simulink model "SignalConditioning_Controller"  (R2021b)
settings: Solver=VariableStepAuto  StartTime=0.0  StopTime=10.0  RelTol=1e-3
settings Model: Creator=matas  LastModifiedBy=matas

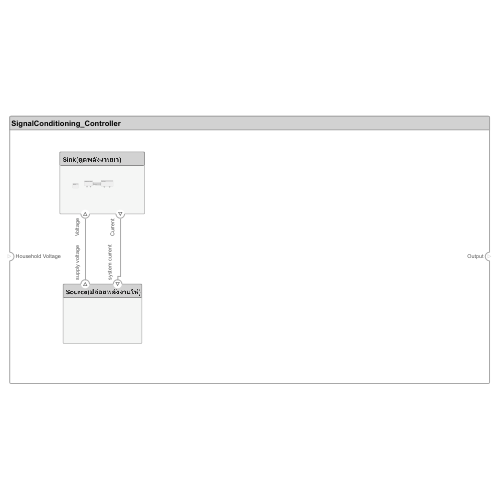
[thumbnail: Simulink's stored preview of the top-level diagram]
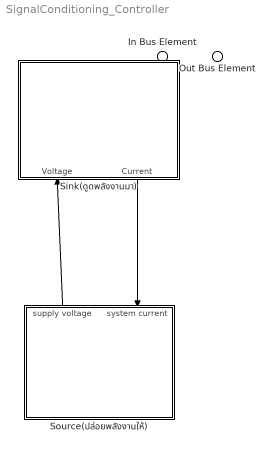
== system SignalConditioning_Controller ==
  In Bus Element : Inport  PortName=Household Voltage
  Sink(ดูดพลังงานมา) : Subsystem
      settings: PortSchema="{\"entries\":[{\"content\":{\"headerSize\":26,\"margin\":15,\"minimumSpacing\":25,\"sides\":[{\"content\":{\"connectorIds\":[]},\"type\":\"ConnectorPlacement.EquallySpacedRectSide\",\"uuid\":\"92879829-3325-4e99-8cb7-644760838beb\"},{\"content\":{\"connectorIds\":[],\"side\":\"RIGHT\"},\"type\":\"ConnectorPlacement.EquallySpacedRectSide\",\"uuid\":\"7f28acab-39b7-45d1-ae7e-3b59846b890e\"},{\"content\":{\"connectorIds\":[],\"side\":\"TOP\"},\"type\":\"ConnectorPlacement.EquallySpacedRectSide\",\"uuid\":\"948d0c2c-a98c-4918-8c8b-513a78882665\"},{\"content\":{\"connectorIds\":[\"In1\",\"Out1\"],\"side\":\"BOTTOM\"},\"type\":\"ConnectorPlacement.EquallySpacedRectSide\",\"uuid\":\"f8beaf20-50aa-47d8-aac6-799df18d83d8\"}]},\"type\":\"ConnectorPlacement.EquallySpacedConnector\",\"uuid\":\"4e812113-efb0-4c93-881b-0cbb00878572\"}],\"packageUris\":[\"http://schema.mathworks.com/mf0/Connector/R2020b\"],\"version\":\"1.0\"}"
  Source(ปล่อยพลังงานให้) : Subsystem
      settings: PortSchema="{\"entries\":[{\"content\":{\"headerSize\":26,\"margin\":15,\"minimumSpacing\":25,\"sides\":[{\"content\":{\"connectorIds\":[]},\"type\":\"ConnectorPlacement.EquallySpacedRectSide\",\"uuid\":\"92879829-3325-4e99-8cb7-644760838beb\"},{\"content\":{\"connectorIds\":[],\"side\":\"RIGHT\"},\"type\":\"ConnectorPlacement.EquallySpacedRectSide\",\"uuid\":\"7f28acab-39b7-45d1-ae7e-3b59846b890e\"},{\"content\":{\"connectorIds\":[\"Out1\",\"In1\"],\"side\":\"TOP\"},\"type\":\"ConnectorPlacement.EquallySpacedRectSide\",\"uuid\":\"948d0c2c-a98c-4918-8c8b-513a78882665\"}]},\"type\":\"ConnectorPlacement.EquallySpacedConnector\",\"uuid\":\"4e812113-efb0-4c93-881b-0cbb00878572\"}],\"packageUris\":[\"http://schema.mathworks.com/mf0/Connector/R2020b\"],\"version\":\"1.0\"}"
  Out Bus Element : Outport  PortName=Output
  wires:
  Source(ปล่อยพลังงานให้)/1(supply voltage) -> Sink(ดูดพลังงานมา)/1(Voltage)
  Sink(ดูดพลังงานมา)/1(Current) -> Source(ปล่อยพลังงานให้)/1(system current)

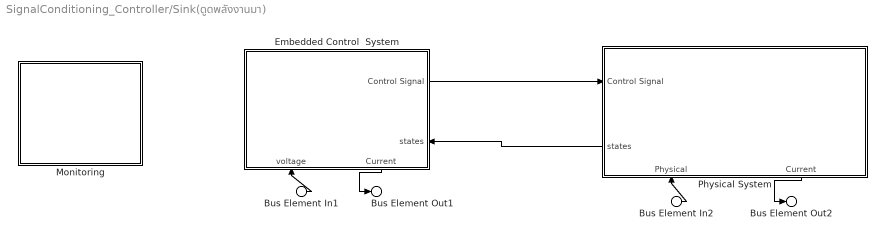
== system SignalConditioning_Controller/Sink(ดูดพลังงานมา) ==
  Bus Element In1 : Inport  PortName=Voltage  Element=Control
  Bus Element In2 : Inport  PortName=Voltage  Element=Physical
  Embedded Control  System : Subsystem
      settings: PortSchema="{\"entries\":[{\"content\":{\"headerSize\":26,\"margin\":15,\"minimumSpacing\":25,\"sides\":[{\"content\":{\"connectorIds\":[]},\"type\":\"ConnectorPlacement.EquallySpacedRectSide\",\"uuid\":\"92879829-3325-4e99-8cb7-644760838beb\"},{\"content\":{\"connectorIds\":[\"Out1\",\"In1\"],\"side\":\"RIGHT\"},\"type\":\"ConnectorPlacement.EquallySpacedRectSide\",\"uuid\":\"7f28acab-39b7-45d1-ae7e-3b59846b890e\"},{\"content\":{\"connectorIds\":[],\"side\":\"TOP\"},\"type\":\"ConnectorPlacement.EquallySpacedRectSide\",\"uuid\":\"948d0c2c-a98c-4918-8c8b-513a78882665\"},{\"content\":{\"connectorIds\":[\"In2\",\"Out2\"],\"side\":\"BOTTOM\"},\"type\":\"ConnectorPlacement.EquallySpacedRectSide\",\"uuid\":\"a92c0028-d905-4fe1-b620-96383c5e960c\"}]},\"type\":\"ConnectorPlacement.EquallySpacedConnector\",\"uuid\":\"4e812113-efb0-4c93-881b-0cbb00878572\"}],\"packageUris\":[\"http://schema.mathworks.com/mf0/Connector/R2020b\"],\"version\":\"1.0\"}"
  Monitoring : Subsystem
      settings: PortSchema="{\"entries\":[{\"content\":{\"headerSize\":26,\"margin\":15,\"minimumSpacing\":25,\"sides\":[{\"content\":{\"connectorIds\":[]},\"type\":\"ConnectorPlacement.EquallySpacedRectSide\",\"uuid\":\"92879829-3325-4e99-8cb7-644760838beb\"},{\"content\":{\"connectorIds\":[],\"side\":\"RIGHT\"},\"type\":\"ConnectorPlacement.EquallySpacedRectSide\",\"uuid\":\"7f28acab-39b7-45d1-ae7e-3b59846b890e\"},{\"content\":{\"connectorIds\":[],\"side\":\"TOP\"},\"type\":\"ConnectorPlacement.EquallySpacedRectSide\",\"uuid\":\"948d0c2c-a98c-4918-8c8b-513a78882665\"}]},\"type\":\"ConnectorPlacement.EquallySpacedConnector\",\"uuid\":\"4e812113-efb0-4c93-881b-0cbb00878572\"}],\"packageUris\":[\"http://schema.mathworks.com/mf0/Connector/R2020b\"],\"version\":\"1.0\"}"
  Physical System : Subsystem
      settings: PortSchema="{\"entries\":[{\"content\":{\"headerSize\":26,\"margin\":15,\"minimumSpacing\":25,\"sides\":[{\"content\":{\"connectorIds\":[\"In1\",\"Out1\"]},\"type\":\"ConnectorPlacement.EquallySpacedRectSide\",\"uuid\":\"92879829-3325-4e99-8cb7-644760838beb\"},{\"content\":{\"connectorIds\":[],\"side\":\"RIGHT\"},\"type\":\"ConnectorPlacement.EquallySpacedRectSide\",\"uuid\":\"7f28acab-39b7-45d1-ae7e-3b59846b890e\"},{\"content\":{\"connectorIds\":[],\"side\":\"TOP\"},\"type\":\"ConnectorPlacement.EquallySpacedRectSide\",\"uuid\":\"948d0c2c-a98c-4918-8c8b-513a78882665\"},{\"content\":{\"connectorIds\":[\"In2\",\"Out2\"],\"side\":\"BOTTOM\"},\"type\":\"ConnectorPlacement.EquallySpacedRectSide\",\"uuid\":\"84b42df1-53ca-4145-9269-aa3d14a2f51f\"}]},\"type\":\"ConnectorPlacement.EquallySpacedConnector\",\"uuid\":\"4e812113-efb0-4c93-881b-0cbb00878572\"}],\"packageUris\":[\"http://schema.mathworks.com/mf0/Connector/R2020b\"],\"version\":\"1.0\"}"
  Bus Element Out1 : Outport  PortName=Current  Element=Control
  Bus Element Out2 : Outport  PortName=Current  Element=Physical
  wires:
  Bus Element In1/1 -> Embedded Control  System/2(voltage)
  Bus Element In2/1 -> Physical System/2(Physical)
  Embedded Control  System/2(Current) -> Bus Element Out1/1
  Physical System/2(Current) -> Bus Element Out2/1
  Embedded Control  System/1(Control Signal) -> Physical System/1(Control Signal)
  Physical System/1(states) -> Embedded Control  System/1(states)

== system SignalConditioning_Controller/Source(ปล่อยพลังงานให้) ==
  Bus Element In1 : Inport  PortName=system current
  Bus Element Out1 : Outport  PortName=supply voltage

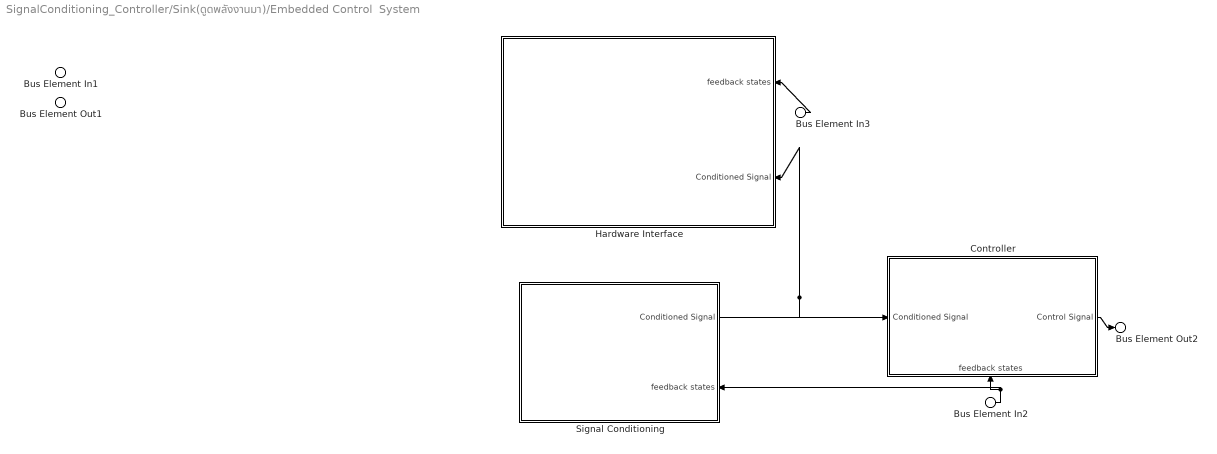
== system SignalConditioning_Controller/Sink(ดูดพลังงานมา)/Embedded Control  System ==
  Bus Element In2 : Inport  PortName=states
  Bus Element In3 : Inport  PortName=states
  Bus Element In1 : Inport  Port=2  PortName=voltage
  Controller : Subsystem
      settings: PortSchema="{\"entries\":[{\"content\":{\"headerSize\":26,\"margin\":15,\"minimumSpacing\":25,\"sides\":[{\"content\":{\"connectorIds\":[\"In2\"]},\"type\":\"ConnectorPlacement.EquallySpacedRectSide\",\"uuid\":\"ceb52414-35d0-489d-844f-0240986ed89c\"},{\"content\":{\"connectorIds\":[\"Out1\"],\"side\":\"RIGHT\"},\"type\":\"ConnectorPlacement.EquallySpacedRectSide\",\"uuid\":\"3638cfe4-de14-450c-b813-3d39c139d6c7\"},{\"content\":{\"connectorIds\":[],\"side\":\"TOP\"},\"type\":\"ConnectorPlacement.EquallySpacedRectSide\",\"uuid\":\"e1a5ba4e-0ffe-4799-9521-abb5e0d1f21a\"},{\"content\":{\"connectorIds\":[\"In1\"],\"side\":\"BOTTOM\"},\"type\":\"ConnectorPlacement.EquallySpacedRectSide\",\"uuid\":\"11d7d3df-85b9-4601-8b25-b97d0b961774\"}]},\"type\":\"ConnectorPlacement.EquallySpacedConnector\",\"uuid\":\"255c5072-1ac3-4228-aa74-c15b1fadc6e8\"}],\"packageUris\":[\"http://schema.mathworks.com/mf0/Connector/R2020b\"],\"version\":\"1.0\"}"
  Hardware Interface : Subsystem
      settings: PortSchema="{\"entries\":[{\"content\":{\"headerSize\":26,\"margin\":15,\"minimumSpacing\":25,\"sides\":[{\"content\":{\"connectorIds\":[]},\"type\":\"ConnectorPlacement.EquallySpacedRectSide\",\"uuid\":\"89c758c6-5bf4-4e3d-884a-0a2d3b628fd4\"},{\"content\":{\"connectorIds\":[\"In1\",\"In2\"],\"side\":\"RIGHT\"},\"type\":\"ConnectorPlacement.EquallySpacedRectSide\",\"uuid\":\"32681a3c-4039-4ddc-888a-6226d07bdd09\"},{\"content\":{\"connectorIds\":[],\"side\":\"TOP\"},\"type\":\"ConnectorPlacement.EquallySpacedRectSide\",\"uuid\":\"9c24464f-60c8-475e-b60e-13d4a1ede9f3\"}]},\"type\":\"ConnectorPlacement.EquallySpacedConnector\",\"uuid\":\"dbaccdc0-8e7e-4e23-bc02-6fb1b571e949\"}],\"packageUris\":[\"http://schema.mathworks.com/mf0/Connector/R2020b\"],\"version\":\"1.0\"}"
  Signal Conditioning : Subsystem
      settings: PortSchema="{\"entries\":[{\"content\":{\"headerSize\":26,\"margin\":15,\"minimumSpacing\":25,\"sides\":[{\"content\":{\"connectorIds\":[]},\"type\":\"ConnectorPlacement.EquallySpacedRectSide\",\"uuid\":\"ec34c04b-13ec-405c-8aad-0b7c99871b48\"},{\"content\":{\"connectorIds\":[\"Out1\",\"In1\"],\"side\":\"RIGHT\"},\"type\":\"ConnectorPlacement.EquallySpacedRectSide\",\"uuid\":\"74d376a0-546b-4ab2-965b-dd49f4bea425\"},{\"content\":{\"connectorIds\":[],\"side\":\"TOP\"},\"type\":\"ConnectorPlacement.EquallySpacedRectSide\",\"uuid\":\"c88818c7-5999-4f33-bb03-6b925a70aaea\"}]},\"type\":\"ConnectorPlacement.EquallySpacedConnector\",\"uuid\":\"6f67766d-4ad9-492c-8b10-a678869122ae\"}],\"packageUris\":[\"http://schema.mathworks.com/mf0/Connector/R2020b\"],\"version\":\"1.0\"}"
  Bus Element Out2 : Outport  PortName=Control Signal
  Bus Element Out1 : Outport  Port=2  PortName=Current
  wires:
  Signal Conditioning/1(Conditioned Signal) -> Hardware Interface/2(Conditioned Signal), Controller/2(Conditioned Signal)
  Controller/1(Control Signal) -> Bus Element Out2/1
  Bus Element In2/1 -> Signal Conditioning/1(feedback states), Controller/1(feedback states)
  Bus Element In3/1 -> Hardware Interface/1(feedback states)

== system SignalConditioning_Controller/Sink(ดูดพลังงานมา)/Monitoring ==

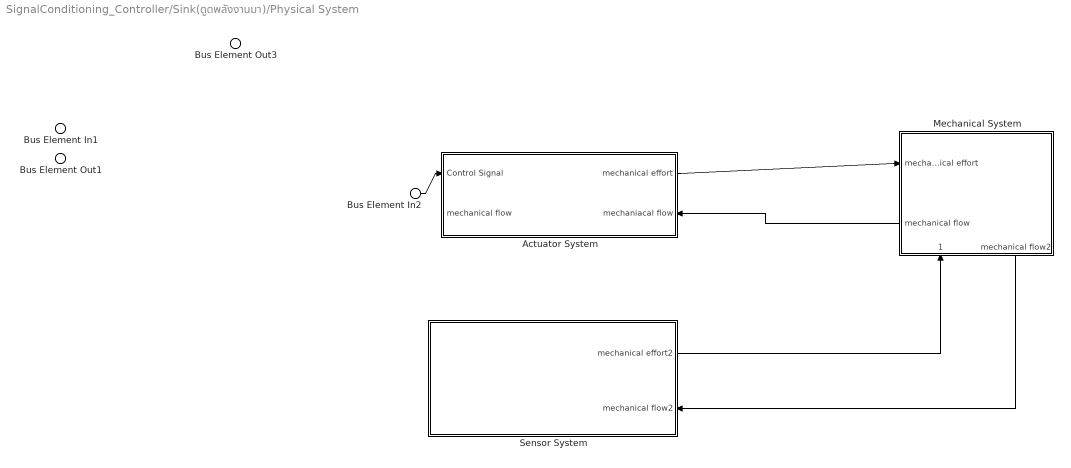
== system SignalConditioning_Controller/Sink(ดูดพลังงานมา)/Physical System ==
  Bus Element In2 : Inport  PortName=Control Signal
  Bus Element In1 : Inport  Port=2  PortName=Physical
  Actuator System : Subsystem
      settings: PortSchema="{\"entries\":[{\"content\":{\"headerSize\":26,\"margin\":15,\"minimumSpacing\":25,\"sides\":[{\"content\":{\"connectorIds\":[\"In2\",\"In3\"]},\"type\":\"ConnectorPlacement.EquallySpacedRectSide\",\"uuid\":\"f68f48cd-d951-4f9c-827f-388e43e3aa01\"},{\"content\":{\"connectorIds\":[\"Out1\",\"In1\"],\"side\":\"RIGHT\"},\"type\":\"ConnectorPlacement.EquallySpacedRectSide\",\"uuid\":\"e5e3824f-74cc-4079-8d6d-75ff73bcf254\"},{\"content\":{\"connectorIds\":[],\"side\":\"TOP\"},\"type\":\"ConnectorPlacement.EquallySpacedRectSide\",\"uuid\":\"cb8d02ba-1207-4662-826d-8ada9ffc348d\"}]},\"type\":\"ConnectorPlacement.EquallySpacedConnector\",\"uuid\":\"3a1957b8-446a-446d-9e0a-16dce487d48a\"}],\"packageUris\":[\"http://schema.mathworks.com/mf0/Connector/R2020b\"],\"version\":\"1.0\"}"
  Mechanical System : Subsystem
      settings: PortSchema="{\"entries\":[{\"content\":{\"headerSize\":26,\"margin\":15,\"minimumSpacing\":25,\"sides\":[{\"content\":{\"connectorIds\":[\"In2\",\"Out2\"]},\"type\":\"ConnectorPlacement.EquallySpacedRectSide\",\"uuid\":\"92879829-3325-4e99-8cb7-644760838beb\"},{\"content\":{\"connectorIds\":[],\"side\":\"RIGHT\"},\"type\":\"ConnectorPlacement.EquallySpacedRectSide\",\"uuid\":\"7f28acab-39b7-45d1-ae7e-3b59846b890e\"},{\"content\":{\"connectorIds\":[],\"side\":\"TOP\"},\"type\":\"ConnectorPlacement.EquallySpacedRectSide\",\"uuid\":\"948d0c2c-a98c-4918-8c8b-513a78882665\"},{\"content\":{\"connectorIds\":[\"In1\",\"Out1\"],\"side\":\"BOTTOM\"},\"type\":\"ConnectorPlacement.EquallySpacedRectSide\",\"uuid\":\"d8e745f5-1ff5-4c8b-af95-de8d750ca6a7\"}]},\"type\":\"ConnectorPlacement.EquallySpacedConnector\",\"uuid\":\"4e812113-efb0-4c93-881b-0cbb00878572\"}],\"packageUris\":[\"http://schema.mathworks.com/mf0/Connector/R2020b\"],\"version\":\"1.0\"}"
  Sensor System : Subsystem
      settings: PortSchema="{\"entries\":[{\"content\":{\"headerSize\":26,\"margin\":15,\"minimumSpacing\":25,\"sides\":[{\"content\":{\"connectorIds\":[]},\"type\":\"ConnectorPlacement.EquallySpacedRectSide\",\"uuid\":\"92879829-3325-4e99-8cb7-644760838beb\"},{\"content\":{\"connectorIds\":[\"Out1\",\"In1\"],\"side\":\"RIGHT\"},\"type\":\"ConnectorPlacement.EquallySpacedRectSide\",\"uuid\":\"7f28acab-39b7-45d1-ae7e-3b59846b890e\"},{\"content\":{\"connectorIds\":[],\"side\":\"TOP\"},\"type\":\"ConnectorPlacement.EquallySpacedRectSide\",\"uuid\":\"948d0c2c-a98c-4918-8c8b-513a78882665\"}]},\"type\":\"ConnectorPlacement.EquallySpacedConnector\",\"uuid\":\"4e812113-efb0-4c93-881b-0cbb00878572\"}],\"packageUris\":[\"http://schema.mathworks.com/mf0/Connector/R2020b\"],\"version\":\"1.0\"}"
  Bus Element Out3 : Outport  PortName=states
  Bus Element Out1 : Outport  Port=2  PortName=Current
  wires:
  Bus Element In2/1 -> Actuator System/2(Control Signal)
  Actuator System/1(mechanical effort) -> Mechanical System/2(mechanical effort)
  Mechanical System/2(mechanical flow) -> Actuator System/1(mechaniacal flow)
  Sensor System/1(mechanical effort2) -> Mechanical System/1(mechanical effort2)
  Mechanical System/1(mechanical flow2) -> Sensor System/1(mechanical flow2)

== system SignalConditioning_Controller/Sink(ดูดพลังงานมา)/Embedded Control  System/Controller ==
  Bus Element In2 : Inport  PortName=feedback states
  Bus Element In1 : Inport  Port=2  PortName=Conditioned Signal
  Bus Element Out1 : Outport  PortName=Control Signal

== system SignalConditioning_Controller/Sink(ดูดพลังงานมา)/Embedded Control  System/Hardware Interface ==
  Bus Element In2 : Inport  PortName=feedback states
  Bus Element In1 : Inport  Port=2  PortName=Conditioned Signal

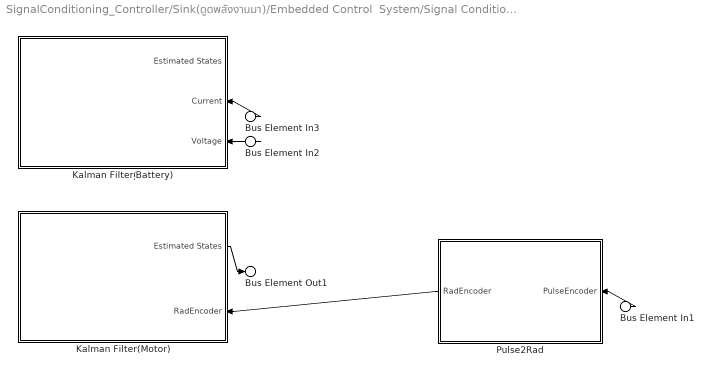
== system SignalConditioning_Controller/Sink(ดูดพลังงานมา)/Embedded Control  System/Signal Conditioning ==
  Bus Element In1 : Inport  PortName=feedback states  Element=PulseEncoder
  Bus Element In2 : Inport  PortName=feedback states  Element=Voltage
  Bus Element In3 : Inport  PortName=feedback states  Element=Current
  Kalman Filter(Motor) : Subsystem
      settings: PortSchema="{\"entries\":[{\"content\":{\"headerSize\":26,\"margin\":15,\"minimumSpacing\":25,\"sides\":[{\"content\":{\"connectorIds\":[]},\"type\":\"ConnectorPlacement.EquallySpacedRectSide\",\"uuid\":\"ec34c04b-13ec-405c-8aad-0b7c99871b48\"},{\"content\":{\"connectorIds\":[\"Out1\",\"In1\"],\"side\":\"RIGHT\"},\"type\":\"ConnectorPlacement.EquallySpacedRectSide\",\"uuid\":\"74d376a0-546b-4ab2-965b-dd49f4bea425\"},{\"content\":{\"connectorIds\":[],\"side\":\"TOP\"},\"type\":\"ConnectorPlacement.EquallySpacedRectSide\",\"uuid\":\"c88818c7-5999-4f33-bb03-6b925a70aaea\"}]},\"type\":\"ConnectorPlacement.EquallySpacedConnector\",\"uuid\":\"6f67766d-4ad9-492c-8b10-a678869122ae\"}],\"packageUris\":[\"http://schema.mathworks.com/mf0/Connector/R2020b\"],\"version\":\"1.0\"}"
  Kalman Filter(ฺBattery) : Subsystem
      settings: PortSchema="{\"entries\":[{\"content\":{\"headerSize\":26,\"margin\":15,\"minimumSpacing\":25,\"sides\":[{\"content\":{\"connectorIds\":[]},\"type\":\"ConnectorPlacement.EquallySpacedRectSide\",\"uuid\":\"ec34c04b-13ec-405c-8aad-0b7c99871b48\"},{\"content\":{\"connectorIds\":[\"Out1\",\"In1\",\"In2\"],\"side\":\"RIGHT\"},\"type\":\"ConnectorPlacement.EquallySpacedRectSide\",\"uuid\":\"74d376a0-546b-4ab2-965b-dd49f4bea425\"},{\"content\":{\"connectorIds\":[],\"side\":\"TOP\"},\"type\":\"ConnectorPlacement.EquallySpacedRectSide\",\"uuid\":\"c88818c7-5999-4f33-bb03-6b925a70aaea\"}]},\"type\":\"ConnectorPlacement.EquallySpacedConnector\",\"uuid\":\"6f67766d-4ad9-492c-8b10-a678869122ae\"}],\"packageUris\":[\"http://schema.mathworks.com/mf0/Connector/R2020b\"],\"version\":\"1.0\"}"
  Pulse2Rad : Subsystem
      settings: PortSchema="{\"entries\":[{\"content\":{\"headerSize\":26,\"margin\":15,\"minimumSpacing\":25,\"sides\":[{\"content\":{\"connectorIds\":[\"Out1\"]},\"type\":\"ConnectorPlacement.EquallySpacedRectSide\",\"uuid\":\"ec34c04b-13ec-405c-8aad-0b7c99871b48\"},{\"content\":{\"connectorIds\":[\"In1\"],\"side\":\"RIGHT\"},\"type\":\"ConnectorPlacement.EquallySpacedRectSide\",\"uuid\":\"74d376a0-546b-4ab2-965b-dd49f4bea425\"},{\"content\":{\"connectorIds\":[],\"side\":\"TOP\"},\"type\":\"ConnectorPlacement.EquallySpacedRectSide\",\"uuid\":\"c88818c7-5999-4f33-bb03-6b925a70aaea\"},{\"content\":{\"connectorIds\":[],\"side\":\"BOTTOM\"},\"type\":\"ConnectorPlacement.EquallySpacedRectSide\",\"uuid\":\"09c25934-beae-47ad-a481-667dee23ffb8\"}]},\"type\":\"ConnectorPlacement.EquallySpacedConnector\",\"uuid\":\"6f67766d-4ad9-492c-8b10-a678869122ae\"}],\"packageUris\":[\"http://schema.mathworks.com/mf0/Connector/R2020b\"],\"version\":\"1.0\"}"
  Bus Element Out1 : Outport  PortName=Conditioned Signal
  wires:
  Bus Element In1/1 -> Pulse2Rad/1(PulseEncoder)
  Pulse2Rad/1(RadEncoder) -> Kalman Filter(Motor)/1(RadEncoder)
  Bus Element In2/1 -> Kalman Filter(ฺBattery)/2(Voltage)
  Bus Element In3/1 -> Kalman Filter(ฺBattery)/1(Current)
  Kalman Filter(Motor)/1(Estimated States) -> Bus Element Out1/1

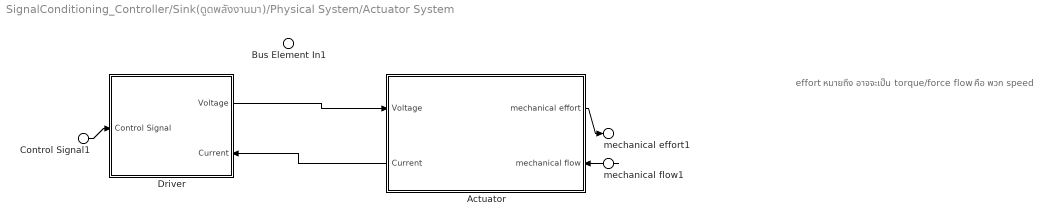
== system SignalConditioning_Controller/Sink(ดูดพลังงานมา)/Physical System/Actuator System ==
  note: effort  หมายถึง อาจจะเป็น torque/force
      | flow คือ พวก speed
  Bus Element In1 : Inport  PortName=mechaniacal flow
  Control Signal1 : Inport  Port=2  PortName=Control Signal
  mechanical flow1 : Inport  Port=3  PortName=mechanical flow
  Actuator : Subsystem
      settings: PortSchema="{\"entries\":[{\"content\":{\"headerSize\":26,\"margin\":15,\"minimumSpacing\":25,\"sides\":[{\"content\":{\"connectorIds\":[\"In2\",\"Out2\"]},\"type\":\"ConnectorPlacement.EquallySpacedRectSide\",\"uuid\":\"92879829-3325-4e99-8cb7-644760838beb\"},{\"content\":{\"connectorIds\":[\"Out1\",\"In1\"],\"side\":\"RIGHT\"},\"type\":\"ConnectorPlacement.EquallySpacedRectSide\",\"uuid\":\"7f28acab-39b7-45d1-ae7e-3b59846b890e\"},{\"content\":{\"connectorIds\":[],\"side\":\"TOP\"},\"type\":\"ConnectorPlacement.EquallySpacedRectSide\",\"uuid\":\"948d0c2c-a98c-4918-8c8b-513a78882665\"}]},\"type\":\"ConnectorPlacement.EquallySpacedConnector\",\"uuid\":\"4e812113-efb0-4c93-881b-0cbb00878572\"}],\"packageUris\":[\"http://schema.mathworks.com/mf0/Connector/R2020b\"],\"version\":\"1.0\"}"
  Driver : Subsystem
      settings: PortSchema="{\"entries\":[{\"content\":{\"headerSize\":26,\"margin\":15,\"minimumSpacing\":25,\"sides\":[{\"content\":{\"connectorIds\":[\"In2\"]},\"type\":\"ConnectorPlacement.EquallySpacedRectSide\",\"uuid\":\"92879829-3325-4e99-8cb7-644760838beb\"},{\"content\":{\"connectorIds\":[\"Out1\",\"In1\"],\"side\":\"RIGHT\"},\"type\":\"ConnectorPlacement.EquallySpacedRectSide\",\"uuid\":\"7f28acab-39b7-45d1-ae7e-3b59846b890e\"},{\"content\":{\"connectorIds\":[],\"side\":\"TOP\"},\"type\":\"ConnectorPlacement.EquallySpacedRectSide\",\"uuid\":\"948d0c2c-a98c-4918-8c8b-513a78882665\"}]},\"type\":\"ConnectorPlacement.EquallySpacedConnector\",\"uuid\":\"4e812113-efb0-4c93-881b-0cbb00878572\"}],\"packageUris\":[\"http://schema.mathworks.com/mf0/Connector/R2020b\"],\"version\":\"1.0\"}"
  mechanical effort1 : Outport  PortName=mechanical effort
  wires:
  Actuator/2(Current) -> Driver/1(Current)
  Driver/1(Voltage) -> Actuator/2(Voltage)
  mechanical flow1/1 -> Actuator/1(mechanical flow)
  Actuator/1(mechanical effort) -> mechanical effort1/1
  Control Signal1/1 -> Driver/2(Control Signal)

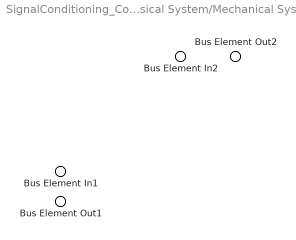
== system SignalConditioning_Controller/Sink(ดูดพลังงานมา)/Physical System/Mechanical System ==
  Bus Element In2 : Inport  PortName=mechanical effort2
  Bus Element In1 : Inport  Port=2  PortName=mechanical effort
  Bus Element Out2 : Outport  PortName=mechanical flow2
  Bus Element Out1 : Outport  Port=2  PortName=mechanical flow

== system SignalConditioning_Controller/Sink(ดูดพลังงานมา)/Physical System/Sensor System ==
  Bus Element In2 : Inport  PortName=mechanical flow2
  Sensors : Subsystem
      settings: PortSchema="{\"entries\":[{\"content\":{\"headerSize\":26,\"margin\":15,\"minimumSpacing\":25,\"sides\":[{\"content\":{\"connectorIds\":[]},\"type\":\"ConnectorPlacement.EquallySpacedRectSide\",\"uuid\":\"92879829-3325-4e99-8cb7-644760838beb\"},{\"content\":{\"connectorIds\":[],\"side\":\"RIGHT\"},\"type\":\"ConnectorPlacement.EquallySpacedRectSide\",\"uuid\":\"7f28acab-39b7-45d1-ae7e-3b59846b890e\"},{\"content\":{\"connectorIds\":[],\"side\":\"TOP\"},\"type\":\"ConnectorPlacement.EquallySpacedRectSide\",\"uuid\":\"948d0c2c-a98c-4918-8c8b-513a78882665\"}]},\"type\":\"ConnectorPlacement.EquallySpacedConnector\",\"uuid\":\"4e812113-efb0-4c93-881b-0cbb00878572\"}],\"packageUris\":[\"http://schema.mathworks.com/mf0/Connector/R2020b\"],\"version\":\"1.0\"}"
  Bus Element Out1 : Outport  PortName=mechanical effort2

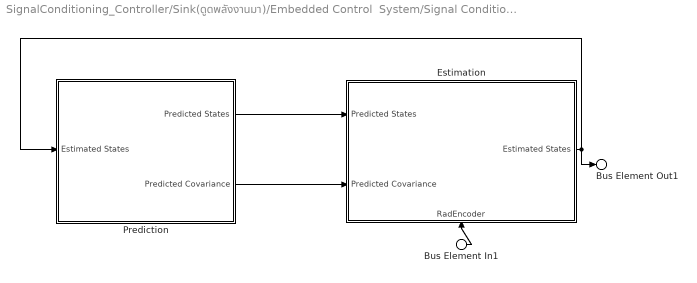
== system SignalConditioning_Controller/Sink(ดูดพลังงานมา)/Embedded Control  System/Signal Conditioning/Kalman Filter(Motor) ==
  Bus Element In1 : Inport  PortName=RadEncoder  Element=Feedback
  Estimation : Subsystem
      settings: PortSchema="{\"entries\":[{\"content\":{\"headerSize\":26,\"margin\":15,\"minimumSpacing\":25,\"sides\":[{\"content\":{\"connectorIds\":[\"In2\",\"In3\"]},\"type\":\"ConnectorPlacement.EquallySpacedRectSide\",\"uuid\":\"ec34c04b-13ec-405c-8aad-0b7c99871b48\"},{\"content\":{\"connectorIds\":[\"Out1\"],\"side\":\"RIGHT\"},\"type\":\"ConnectorPlacement.EquallySpacedRectSide\",\"uuid\":\"74d376a0-546b-4ab2-965b-dd49f4bea425\"},{\"content\":{\"connectorIds\":[],\"side\":\"TOP\"},\"type\":\"ConnectorPlacement.EquallySpacedRectSide\",\"uuid\":\"c88818c7-5999-4f33-bb03-6b925a70aaea\"},{\"content\":{\"connectorIds\":[\"In1\"],\"side\":\"BOTTOM\"},\"type\":\"ConnectorPlacement.EquallySpacedRectSide\",\"uuid\":\"14be066e-5bbf-4d48-9dcc-1180602027c2\"}]},\"type\":\"ConnectorPlacement.EquallySpacedConnector\",\"uuid\":\"6f67766d-4ad9-492c-8b10-a678869122ae\"}],\"packageUris\":[\"http://schema.mathworks.com/mf0/Connector/R2020b\"],\"version\":\"1.0\"}"
  Prediction : Subsystem
      settings: PortSchema="{\"entries\":[{\"content\":{\"headerSize\":26,\"margin\":15,\"minimumSpacing\":25,\"sides\":[{\"content\":{\"connectorIds\":[\"In1\"]},\"type\":\"ConnectorPlacement.EquallySpacedRectSide\",\"uuid\":\"ec34c04b-13ec-405c-8aad-0b7c99871b48\"},{\"content\":{\"connectorIds\":[\"Out1\",\"Out2\"],\"side\":\"RIGHT\"},\"type\":\"ConnectorPlacement.EquallySpacedRectSide\",\"uuid\":\"74d376a0-546b-4ab2-965b-dd49f4bea425\"},{\"content\":{\"connectorIds\":[],\"side\":\"TOP\"},\"type\":\"ConnectorPlacement.EquallySpacedRectSide\",\"uuid\":\"c88818c7-5999-4f33-bb03-6b925a70aaea\"}]},\"type\":\"ConnectorPlacement.EquallySpacedConnector\",\"uuid\":\"6f67766d-4ad9-492c-8b10-a678869122ae\"}],\"packageUris\":[\"http://schema.mathworks.com/mf0/Connector/R2020b\"],\"version\":\"1.0\"}"
  Bus Element Out1 : Outport  PortName=Estimated States
  wires:
  Prediction/1(Predicted States) -> Estimation/2(Predicted States)
  Estimation/1(Estimated States) -> Prediction/1(Estimated States), Bus Element Out1/1
  Prediction/2(Predicted Covariance) -> Estimation/3(Predicted Covariance)
  Bus Element In1/1 -> Estimation/1(RadEncoder)

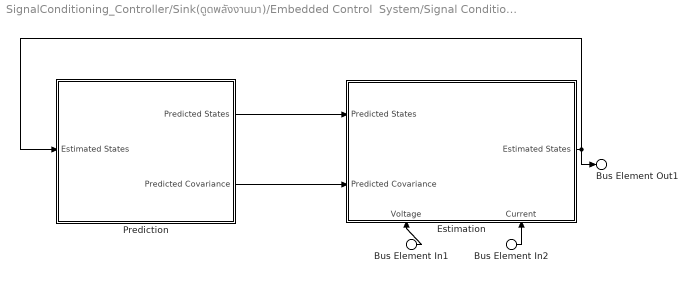
== system SignalConditioning_Controller/Sink(ดูดพลังงานมา)/Embedded Control  System/Signal Conditioning/Kalman Filter(ฺBattery) ==
  Bus Element In2 : Inport  PortName=Current  Element=Feedback
  Bus Element In1 : Inport  Port=2  PortName=Voltage  Element=Feedback
  Estimation : Subsystem
      settings: PortSchema="{\"entries\":[{\"content\":{\"headerSize\":26,\"margin\":15,\"minimumSpacing\":25,\"sides\":[{\"content\":{\"connectorIds\":[\"In3\",\"In4\"]},\"type\":\"ConnectorPlacement.EquallySpacedRectSide\",\"uuid\":\"ec34c04b-13ec-405c-8aad-0b7c99871b48\"},{\"content\":{\"connectorIds\":[\"Out1\"],\"side\":\"RIGHT\"},\"type\":\"ConnectorPlacement.EquallySpacedRectSide\",\"uuid\":\"74d376a0-546b-4ab2-965b-dd49f4bea425\"},{\"content\":{\"connectorIds\":[],\"side\":\"TOP\"},\"type\":\"ConnectorPlacement.EquallySpacedRectSide\",\"uuid\":\"c88818c7-5999-4f33-bb03-6b925a70aaea\"},{\"content\":{\"connectorIds\":[\"In1\",\"In2\"],\"side\":\"BOTTOM\"},\"type\":\"ConnectorPlacement.EquallySpacedRectSide\",\"uuid\":\"14be066e-5bbf-4d48-9dcc-1180602027c2\"}]},\"type\":\"ConnectorPlacement.EquallySpacedConnector\",\"uuid\":\"6f67766d-4ad9-492c-8b10-a678869122ae\"}],\"packageUris\":[\"http://schema.mathworks.com/mf0/Connector/R2020b\"],\"version\":\"1.0\"}"
  Prediction : Subsystem
      settings: PortSchema="{\"entries\":[{\"content\":{\"headerSize\":26,\"margin\":15,\"minimumSpacing\":25,\"sides\":[{\"content\":{\"connectorIds\":[\"In1\"]},\"type\":\"ConnectorPlacement.EquallySpacedRectSide\",\"uuid\":\"ec34c04b-13ec-405c-8aad-0b7c99871b48\"},{\"content\":{\"connectorIds\":[\"Out1\",\"Out2\"],\"side\":\"RIGHT\"},\"type\":\"ConnectorPlacement.EquallySpacedRectSide\",\"uuid\":\"74d376a0-546b-4ab2-965b-dd49f4bea425\"},{\"content\":{\"connectorIds\":[],\"side\":\"TOP\"},\"type\":\"ConnectorPlacement.EquallySpacedRectSide\",\"uuid\":\"c88818c7-5999-4f33-bb03-6b925a70aaea\"}]},\"type\":\"ConnectorPlacement.EquallySpacedConnector\",\"uuid\":\"6f67766d-4ad9-492c-8b10-a678869122ae\"}],\"packageUris\":[\"http://schema.mathworks.com/mf0/Connector/R2020b\"],\"version\":\"1.0\"}"
  Bus Element Out1 : Outport  PortName=Estimated States
  wires:
  Prediction/1(Predicted States) -> Estimation/3(Predicted States)
  Estimation/1(Estimated States) -> Prediction/1(Estimated States), Bus Element Out1/1
  Prediction/2(Predicted Covariance) -> Estimation/4(Predicted Covariance)
  Bus Element In1/1 -> Estimation/1(Voltage)
  Bus Element In2/1 -> Estimation/2(Current)

== system SignalConditioning_Controller/Sink(ดูดพลังงานมา)/Embedded Control  System/Signal Conditioning/Pulse2Rad ==
  Bus Element In1 : Inport  PortName=PulseEncoder
  Bus Element Out1 : Outport  PortName=RadEncoder

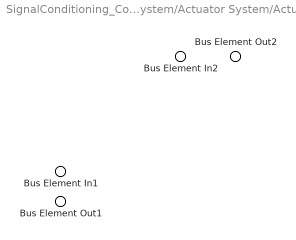
== system SignalConditioning_Controller/Sink(ดูดพลังงานมา)/Physical System/Actuator System/Actuator ==
  Bus Element In2 : Inport  PortName=mechanical flow
  Bus Element In1 : Inport  Port=2  PortName=Voltage
  Bus Element Out2 : Outport  PortName=mechanical effort
  Bus Element Out1 : Outport  Port=2  PortName=Current

== system SignalConditioning_Controller/Sink(ดูดพลังงานมา)/Physical System/Actuator System/Driver ==
  Bus Element In2 : Inport  PortName=Current
  Bus Element In1 : Inport  Port=2  PortName=Control Signal
  Bus Element Out1 : Outport  PortName=Voltage

== system SignalConditioning_Controller/Sink(ดูดพลังงานมา)/Physical System/Sensor System/Sensors ==

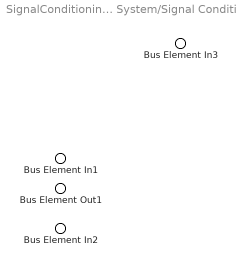
== system SignalConditioning_Controller/Sink(ดูดพลังงานมา)/Embedded Control  System/Signal Conditioning/Kalman Filter(Motor)/Estimation ==
  Bus Element In3 : Inport  PortName=RadEncoder
  Bus Element In1 : Inport  Port=2  PortName=Predicted States
  Bus Element In2 : Inport  Port=3  PortName=Predicted Covariance
  Bus Element Out1 : Outport  PortName=Estimated States

== system SignalConditioning_Controller/Sink(ดูดพลังงานมา)/Embedded Control  System/Signal Conditioning/Kalman Filter(Motor)/Prediction ==
  Bus Element In1 : Inport  PortName=Estimated States
  Bus Element Out1 : Outport  PortName=Predicted States
  Bus Element Out2 : Outport  Port=2  PortName=Predicted Covariance

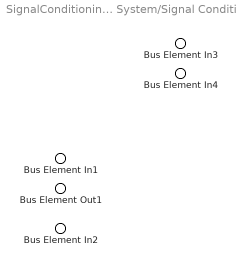
== system SignalConditioning_Controller/Sink(ดูดพลังงานมา)/Embedded Control  System/Signal Conditioning/Kalman Filter(ฺBattery)/Estimation ==
  Bus Element In3 : Inport  PortName=Voltage
  Bus Element In4 : Inport  Port=2  PortName=Current
  Bus Element In1 : Inport  Port=3  PortName=Predicted States
  Bus Element In2 : Inport  Port=4  PortName=Predicted Covariance
  Bus Element Out1 : Outport  PortName=Estimated States

== system SignalConditioning_Controller/Sink(ดูดพลังงานมา)/Embedded Control  System/Signal Conditioning/Kalman Filter(ฺBattery)/Prediction ==
  Bus Element In1 : Inport  PortName=Estimated States
  Bus Element Out1 : Outport  PortName=Predicted States
  Bus Element Out2 : Outport  Port=2  PortName=Predicted Covariance
